simulink model "guide_system"  (R2019b)
settings: Solver=FixedStepAuto  StartTime=0.0  StopTime=450  FixedStep=0.1  RelTol=1e-3
libraries: simulink_need_slupdate x1, simulink x1
settings Model: Creator=Zhexuanx  LastModifiedBy=nguyenhd
settings DataIOCC: ReturnWorkspaceOutputs=off
settings DebuggingCC: ArithmeticOperatorsInVariantConditions=warning
settings SFSimCC: SimUseLocalCustomCode=off  CustomCodeUndefinedFunction=UseInterfaceOnly
settings RTWCC: RTWUseLocalCustomCode=off

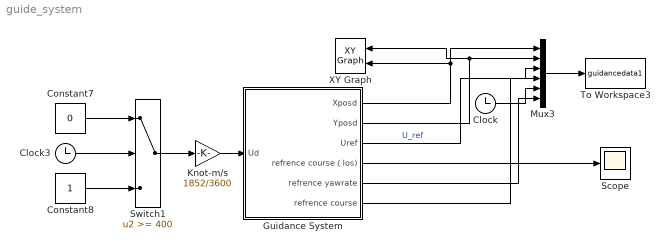
== system guide_system ==
  Clock : Clock
  Clock3 : Clock
  Constant7 : Constant  Value=0
  Constant8 : Constant
  Guidance System : Subsystem
  Knot-m/s : Gain  Gain=1852/3600  SaturateOnIntegerOverflow=on  OutDataTypeStr=Inherit: Same as input  ParamDataTypeStr=Inherit: Same as input
  Mux3 : Mux  Inputs=6
  Scope : Scope
  Switch1 : Switch  Threshold=400  SaturateOnIntegerOverflow=on  InputSameDT=on
  To Workspace3 : ToWorkspace  VariableName=guidancedata1  SampleTime=-1
      settings: Decimation=2
  XY Graph : simulink/Sinks/XY Graph  xmin=-100  xmax=300  ymin=-10  ymax=100  st=-1
  wires:
  Constant8/1 -> Switch1/3
  Switch1/1 -> Knot-m/s/1
  Clock3/1 -> Switch1/2
  Guidance System/1(Xposd) -> XY Graph/2, Mux3/1
  Constant7/1 -> Switch1/1
  Knot-m/s/1 -> Guidance System/1(Ud)
  Guidance System/2(Yposd) -> XY Graph/1, Mux3/2
  Guidance System/4(refrence course（los)) -> Scope/1
  Clock/1 -> Mux3/5
  Guidance System/6(refrence course) -> Mux3/4
  Mux3/1 -> To Workspace3/1
  Guidance System/3(Uref) -> Mux3/3  "U_ref"
  Guidance System/5(refrence yawrate) -> Mux3/6

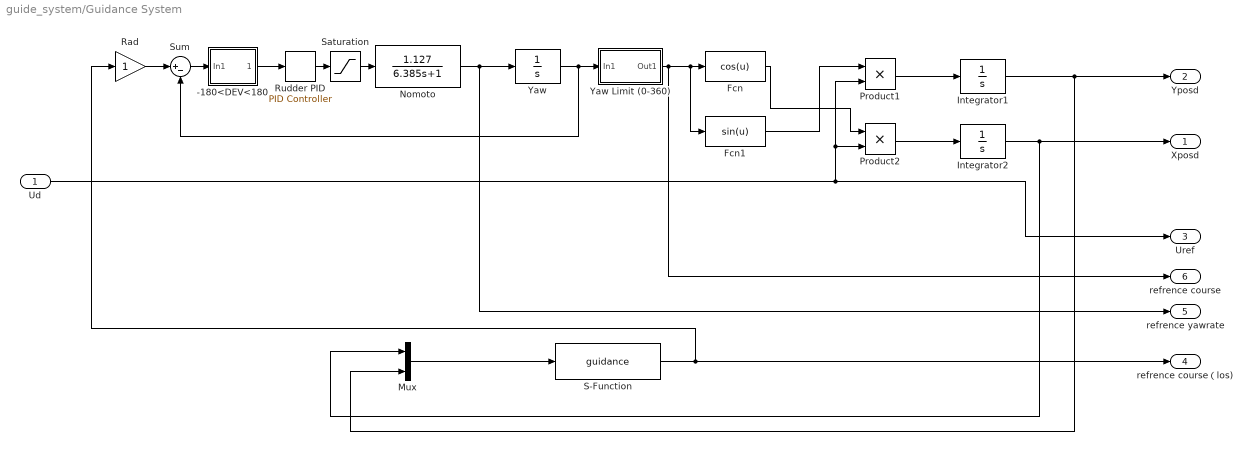
== system guide_system/Guidance System ==
  Ud : Inport
  -180<DEV<180 : Subsystem
  Fcn : Fcn  Expr=cos(u)
  Fcn1 : Fcn  Expr=sin(u)
  Integrator1 : Integrator
  Integrator2 : Integrator
  Mux : Mux  Inputs=2
  Nomoto : TransferFcn  Numerator=[1.127]  Denominator=[6.385 1]
  Product1 : Product  SaturateOnIntegerOverflow=on  RndMeth=Zero  InputSameDT=on  OutDataTypeStr=Inherit: Same as first input
  Product2 : Product  SaturateOnIntegerOverflow=on  RndMeth=Zero  InputSameDT=on  OutDataTypeStr=Inherit: Same as first input
  Rad : Gain  SaturateOnIntegerOverflow=on  OutDataTypeStr=Inherit: Same as input  ParamDataTypeStr=Inherit: Same as input
  Rudder PID : simulink_need_slupdate/PID Controller  P=0.4  I=0  D=4
      settings: SourceProductName=Simulink
  S-Function : S-Function  FunctionName=guidance  SFunctionDeploymentMode=off  EnableBusSupport=off
  Saturation : Saturate  UpperLimit=40*pi/180  LowerLimit=-40*pi/180
  Sum : Sum  Inputs=|+-  SaturateOnIntegerOverflow=on  InputSameDT=on  OutDataTypeStr=Inherit: Same as first input
  Yaw : Integrator  InitialCondition=90*pi/180
  Yaw Limit (0-360) : Subsystem
  Xposd : Outport  VectorParamsAs1DForOutWhenUnconnected=off
  Yposd : Outport  Port=2  VectorParamsAs1DForOutWhenUnconnected=off
  Uref : Outport  Port=3  VectorParamsAs1DForOutWhenUnconnected=off
  refrence course（los) : Outport  Port=4  VectorParamsAs1DForOutWhenUnconnected=off
  refrence yawrate : Outport  Port=5  VectorParamsAs1DForOutWhenUnconnected=off
  refrence course : Outport  Port=6  VectorParamsAs1DForOutWhenUnconnected=off
  wires:
  Sum/1 -> -180<DEV<180/1(In1)
  Fcn/1 -> Product2/1
  Fcn1/1 -> Product1/1
  Product1/1 -> Integrator1/1
  Product2/1 -> Integrator2/1
  Mux/1 -> S-Function/1
  Integrator1/1 -> Mux/2, Yposd/1
  Integrator2/1 -> Mux/1, Xposd/1
  Yaw/1 -> Sum/2, Yaw Limit (0-360)/1(In1)
  Rad/1 -> Sum/1
  S-Function/1 -> Rad/1, refrence course（los)/1
  Nomoto/1 -> refrence yawrate/1, Yaw/1
  Ud/1 -> Product1/2, Product2/2, Uref/1
  Yaw Limit (0-360)/1(Out1) -> refrence course/1, Fcn/1, Fcn1/1
  -180<DEV<180/1(Out1) -> Rudder PID/1
  Rudder PID/1 -> Saturation/1
  Saturation/1 -> Nomoto/1

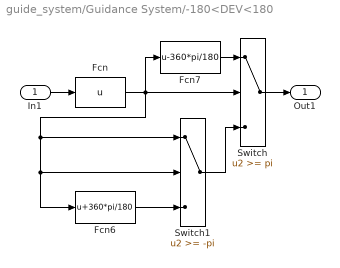
== system guide_system/Guidance System/-180<DEV<180 ==
  In1 : Inport
  Fcn : Fcn  Expr=u
  Fcn6 : Fcn  Expr=u+360*pi/180
  Fcn7 : Fcn  Expr=u-360*pi/180
  Switch : Switch  Threshold=pi  SaturateOnIntegerOverflow=on  InputSameDT=on
  Switch1 : Switch  Threshold=-pi  SaturateOnIntegerOverflow=on  InputSameDT=on
  Out1 : Outport  InitialOutput=0  VectorParamsAs1DForOutWhenUnconnected=off
  wires:
  Fcn/1 -> Switch/2, Switch1/1, Fcn6/1, Switch1/2, Fcn7/1
  In1/1 -> Fcn/1
  Switch/1 -> Out1/1
  Fcn7/1 -> Switch/1
  Fcn6/1 -> Switch1/3
  Switch1/1 -> Switch/3

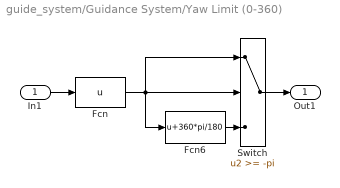
== system guide_system/Guidance System/Yaw Limit (0-360) ==
  In1 : Inport
  Fcn : Fcn  Expr=u
  Fcn6 : Fcn  Expr=u+360*pi/180
  Switch : Switch  Threshold=-pi  SaturateOnIntegerOverflow=on  InputSameDT=on
  Out1 : Outport  InitialOutput=0  VectorParamsAs1DForOutWhenUnconnected=off
  wires:
  Switch/1 -> Out1/1
  In1/1 -> Fcn/1
  Fcn/1 -> Switch/1, Fcn6/1, Switch/2
  Fcn6/1 -> Switch/3
